simulink model "mult35x35_tb"  (Simulink 6.6)
settings: Solver=ode45  StartTime=0.0  StopTime=1000  RelTol=1e-3
undefined symbols (not defined in the file): A, B
libraries: xbsIndex_r4 x168, simulink x2, xbsCopyrightNotice_r4 x1
(part 2 of 2)

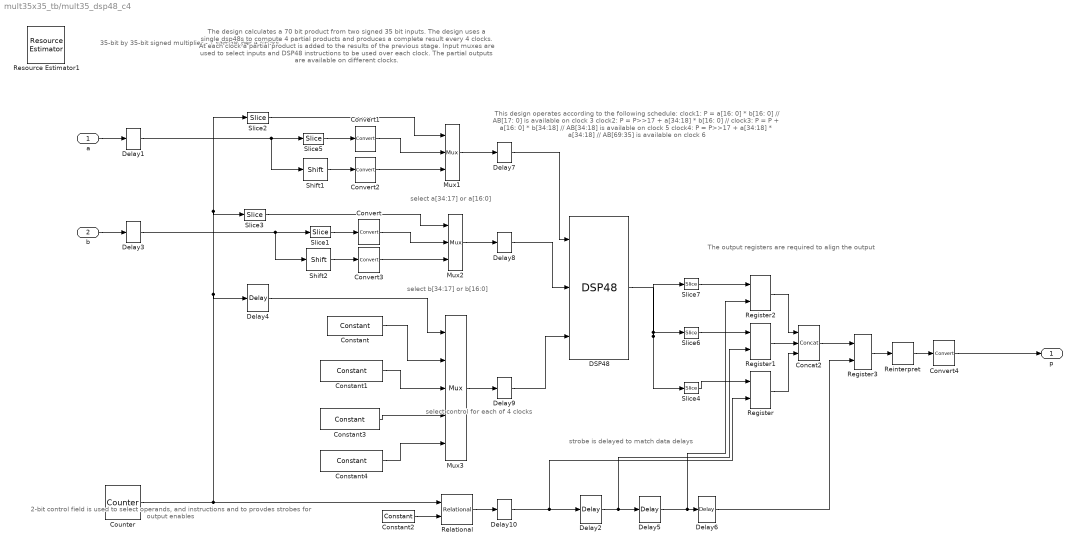
== system mult35x35_tb/mult35_dsp48_c4 ==
  note: select a[34:17] or a[16:0]
  note: 35-bit by 35-bit signed multiplier -
      | 1 sample per 4 clocks
  note: This design operates according to the following schedule:
      |
      | clock1: P =           a[16: 0] * b[16: 0] // AB[17: 0] is available on clock 3
      | clock2: P = P>>17  +  a[34:18] * b[16: 0] //
      | clock3: P = P      +  a[16: 0] * b[34:18] // AB[34:18] is available on clock 5
      | clock4: P = P>>17  +  a[34:18] * a[34:18] // AB[69:35] is available on clock 6
  note: select b[34:17] or b[16:0]
  note: select control for each of 4 clocks
  note: 2-bit control field is used to select operands,
      | and instructions and to provdes strobes for output enables
  note: The design calculates a 70 bit product from two signed 35 bit inputs.
      | The design uses a single  dsp48s to compute 4 partial products and produces a complete result every 4 clocks.
      | At each clock a partial product is added to the results of the previous stage. Input muxes are used to select inputs
      | and DSP48 instructions to be used over each clock. The partial outputs are available on different clocks.
  note: The output registers are required to align the output
  note: strobe is delayed to match data delays
  a : Inport
  b : Inport  Port=2
  Concat2 : xbsIndex_r4/Concat  num_inputs=3  dbl_ovrd=off  block_type=concat
      settings: block_version=VER_STRING_GOES_HERE
  Constant : xbsIndex_r4/Constant  arith_type=DSP48 Instruction  const=1  n_bits=1  bin_pt=0  explicit_period=off  period=1  equ=P=+A*B  opselect=A * B  inp2=PCIN>>17  opr=+  inp1=P  carry=CIN  dbl_ovrd=off  block_type=constant
      settings: block_version=VER_STRING_GOES_HERE
  Constant1 : xbsIndex_r4/Constant  arith_type=DSP48 Instruction  const=1  n_bits=1  bin_pt=0  explicit_period=off  period=1  equ=P=P>>17+(A*B)  opselect=Custom  inp2=P>>17  opr=+  inp1=A*B  carry=0  dbl_ovrd=off  block_type=constant
      settings: block_version=VER_STRING_GOES_HERE
  Constant2 : xbsIndex_r4/Constant  arith_type=Unsigned  const=3  n_bits=2  bin_pt=0  explicit_period=off  period=1  equ=P=C  opselect=C  inp2=PCIN>>17  opr=+  inp1=P  carry=CIN  dbl_ovrd=off  block_type=constant
      settings: block_version=VER_STRING_GOES_HERE
  Constant3 : xbsIndex_r4/Constant  arith_type=DSP48 Instruction  const=1  n_bits=1  bin_pt=0  explicit_period=off  period=1  equ=P=P+(A*B)  opselect=Custom  inp2=P  opr=+  inp1=A*B  carry=0  dbl_ovrd=off  block_type=constant
      settings: block_version=VER_STRING_GOES_HERE
  Constant4 : xbsIndex_r4/Constant  arith_type=DSP48 Instruction  const=1  n_bits=1  bin_pt=0  explicit_period=off  period=1  equ=P=P>>17+(A*B)  opselect=Custom  inp2=P>>17  opr=+  inp1=A*B  carry=0  dbl_ovrd=off  block_type=constant
      settings: block_version=VER_STRING_GOES_HERE
  Convert{,1..3} (4 alike) : xbsIndex_r4/Convert  arith_type="Signed  (2's comp)"  n_bits=18  bin_pt=0  quantization=Truncate  overflow=Wrap  latency=0  dbl_ovrd=off  pipeline=off  block_type=convert
      settings: infoedit=The input is presented at the output after quantization and overflow effects.<P><P>Hardware notes: Additional hardware is used when rounding or saturation is selected and output width is less than the input width.  xl_area=[0 0 0 0 0 0 0]  block_version=VER_STRING_GOES_HERE
  Convert4 : xbsIndex_r4/Convert  arith_type="Signed  (2's comp)"  n_bits=71  bin_pt=0  quantization=Truncate  overflow=Wrap  latency=0  dbl_ovrd=off  pipeline=off  block_type=convert
      settings: infoedit=The input is presented at the output after quantization and overflow effects.<P><P>Hardware notes: Additional hardware is used when rounding or saturation is selected and output width is less than the input width.  xl_area=[0 0 0 0 0 0 0]  block_version=VER_STRING_GOES_HERE
  Counter : xbsIndex_r4/Counter  cnt_type=Free Running  cnt_to=Inf  operation=Up  start_count=0  cnt_by_val=1  arith_type=Unsigned  n_bits=2  bin_pt=0  load_pin=off  rst=off  en=off  explicit_period=on  period=1  dbl_ovrd=off  use_behavioral_HDL=on  use_rpm=off  block_type=counter
      settings: infoedit="Configurable up, down and up/down counter.<P><P>Hardware notes: Free running counters are the least expensive in hardware.  A count limited counter is implemented by combining a counter with a comparator."  xl_area=[1 2 0 2 0 0 0]  block_version=VER_STRING_GOES_HERE
  DSP48 : xbsIndex_r4/DSP48  use_b=Direct from B Port  use_op=on  use_creg=off  use_pcin=off  use_pcout=off  use_bcout=off  rst_all=off  en_all=off  pipeline_a=1  pipeline_b=1  pipeline_c=on  pipeline_p=on  pipeline_mult=on  pipeline_opmode=on  pipeline_sub=on  pipeline_carryin=on  pipeline_carryinsel=on  rst_a=off  rst_b=off  rst_c=off  rst_mult=off  rst_p=off  rst_carry_in=off  rst_ctrl=off  en_a=off  en_b=off  en_c=off  en_mult=off  en_p=off  en_carry_in=off  en_ctrl=off  dbl_ovrd=off  use_synth_model=off  xl_useadderonly=off  block_type=dsp48
      settings: xl_use_area=on  xl_area=[0, 0, 0, 0, 0, 0, 0]  block_version=VER_STRING_GOES_HERE
  Delay{1,3..10} (9 alike) : xbsIndex_r4/Delay  en=off  latency=1  dbl_ovrd=off  reg_retiming=off  block_type=delay
      Delay1 settings: infoedit="Delay line having  configurable length.<P><P>Hardware notes: A delay line is a chain, each link of which is an SRL16 followed by a flip-flop. If register retiming is enabled, the delay line is a chain of flip-flops."  xl_area=[1 1 0 0 0 0 0]  block_version=VER_STRING_GOES_HERE
      Delay10 settings: infoedit="Delay line having  configurable length.<P><P>Hardware notes: A delay line is a chain, each link of which is an SRL16 followed by a flip-flop. If register retiming is enabled, the delay line is a chain of flip-flops."  xl_area=[1 1 0 0 0 0 0]  block_version=VER_STRING_GOES_HERE
      Delay3 settings: infoedit="Delay line having  configurable length.<P><P>Hardware notes: A delay line is a chain, each link of which is an SRL16 followed by a flip-flop. If register retiming is enabled, the delay line is a chain of flip-flops."  xl_area=[1 1 0 0 0 0 0]  block_version=VER_STRING_GOES_HERE
      Delay4 settings: infoedit="Delay line having  configurable length.<P><P>Hardware notes: A delay line is a chain, each link of which is an SRL16 followed by a flip-flop. If register retiming is enabled, the delay line is a chain of flip-flops."  xl_area=[1 2 0 0 0 0 0]  block_version=VER_STRING_GOES_HERE
      Delay5 settings: infoedit="Delay line having  configurable length.<P><P>Hardware notes: A delay line is a chain, each link of which is an SRL16 followed by a flip-flop. If register retiming is enabled, the delay line is a chain of flip-flops."  xl_area=[1 1 0 0 0 0 0]  block_version=VER_STRING_GOES_HERE
      Delay6 settings: infoedit="Delay line having  configurable length.<P><P>Hardware notes: A delay line is a chain, each link of which is an SRL16 followed by a flip-flop. If register retiming is enabled, the delay line is a chain of flip-flops."  xl_area=[1 1 0 0 0 0 0]  block_version=VER_STRING_GOES_HERE
      Delay7 settings: infoedit="Delay line having  configurable length.<P><P>Hardware notes: A delay line is a chain, each link of which is an SRL16 followed by a flip-flop. If register retiming is enabled, the delay line is a chain of flip-flops."  xl_area=[1 1 0 0 0 0 0]  block_version=VER_STRING_GOES_HERE
      Delay8 settings: infoedit="Delay line having  configurable length.<P><P>Hardware notes: A delay line is a chain, each link of which is an SRL16 followed by a flip-flop. If register retiming is enabled, the delay line is a chain of flip-flops."  xl_area=[1 1 0 0 0 0 0]  block_version=VER_STRING_GOES_HERE
      Delay9 settings: infoedit="Delay line having  configurable length.<P><P>Hardware notes: A delay line is a chain, each link of which is an SRL16 followed by a flip-flop. If register retiming is enabled, the delay line is a chain of flip-flops."  xl_area=[1 1 0 0 0 0 0]  block_version=VER_STRING_GOES_HERE
  Delay2 : xbsIndex_r4/Delay  en=off  latency=2  dbl_ovrd=off  reg_retiming=off  block_type=delay
      settings: infoedit="Delay line having  configurable length.<P><P>Hardware notes: A delay line is a chain, each link of which is an SRL16 followed by a flip-flop. If register retiming is enabled, the delay line is a chain of flip-flops."  xl_area=[1 1 0 1 0 0 0]  block_version=VER_STRING_GOES_HERE
  Mux1 : xbsIndex_r4/Mux  inputs=2  en=off  latency=0  precision=Full  arith_type=Unsigned  n_bits=48  bin_pt=0  quantization=Truncate  overflow=Wrap  dbl_ovrd=off  block_type=mux
      settings: xl_area=[9 0 0 18 0 0 0]  block_version=VER_STRING_GOES_HERE
  Mux2 : xbsIndex_r4/Mux  inputs=2  en=off  latency=0  precision=Full  arith_type=Unsigned  n_bits=48  bin_pt=0  quantization=Truncate  overflow=Wrap  dbl_ovrd=off  block_type=mux
      settings: xl_area=[9 0 0 18 0 0 0]  block_version=VER_STRING_GOES_HERE
  Mux3 : xbsIndex_r4/Mux  inputs=4  en=off  latency=0  precision=Full  arith_type=Unsigned  n_bits=48  bin_pt=0  quantization=Truncate  overflow=Wrap  dbl_ovrd=off  block_type=mux
      settings: xl_area=[11 0 0 22 0 0 0]  block_version=VER_STRING_GOES_HERE
  Register{,1..3} (4 alike) : xbsIndex_r4/Register  init=0  rst=off  en=on  dbl_ovrd=off  block_type=register
      Register settings: xl_area=[9 17 0 0 0 0 0]  block_version=VER_STRING_GOES_HERE
      Register1 settings: xl_area=[9 17 0 0 0 0 0]  block_version=VER_STRING_GOES_HERE
      Register2 settings: xl_area=[18 36 0 0 0 0 0]  block_version=VER_STRING_GOES_HERE
      Register3 settings: xl_area=[35 70 0 0 0 0 0]  block_version=VER_STRING_GOES_HERE
  Reinterpret : xbsIndex_r4/Reinterpret  force_arith_type=on  arith_type="Signed  (2's comp)"  force_bin_pt=on  bin_pt=0  block_type=cast
      settings: infoedit="Changes type of samples without altering their binary representation.<P><P>Hardware notes: In hardware this block costs nothing.<P><P>Example:  Suppose the input is 6 bits wide, signed, with 2 fractional bits, and the output is forced to unsigned with 0 fractional bits.  Then an input of -2.0 (1110.00 in binary 2's complement) becomes an output of 56 (111000 in binary)."  block_version=VER_STRING_GOES_HERE
  Relational : xbsIndex_r4/Relational  mode=a=b  en=off  latency=0  dbl_ovrd=off  block_type=relational
      settings: xl_area=[1 0 0 1 0 0 0]  block_version=VER_STRING_GOES_HERE
  Resource Estimator1 : xbsIndex_r4/Resource Estimator  Tag=resEstTag  Slices=896  FFs=1554  BRAMs=0  LUTs=775  IOBs=545  EBMs=8  TBUFs=0  xl_use_estimator_area=off  est_options=Estimate  xl_estimator_area=[896 1554 0 775 545 8 0]  mrp_directory=I:\sg48\src  simulink_period=1/16  block_type=resource_estimator
      settings: AttributesFormatString=Resource\nEstimator  block_version=9.2.00
  Shift1 : xbsIndex_r4/Shift  shift_dir=Right  shift_bits=17  en=off  latency=0  precision=Full  arith_type="Signed  (2's comp)"  n_bits=8  bin_pt=2  quantization=Truncate  overflow=Wrap  dbl_ovrd=off  block_type=shift
      settings: xl_area=[0 0 0 0 0 0 0]  block_version=VER_STRING_GOES_HERE
  Shift2 : xbsIndex_r4/Shift  shift_dir=Right  shift_bits=17  en=off  latency=0  precision=Full  arith_type="Signed  (2's comp)"  n_bits=8  bin_pt=2  quantization=Truncate  overflow=Wrap  dbl_ovrd=off  block_type=shift
      settings: xl_area=[0 0 0 0 0 0 0]  block_version=VER_STRING_GOES_HERE
  Slice{1,4..6} (4 alike) : xbsIndex_r4/Slice  nbits=17  boolean_output=off  mode=Lower Bit Location + Width  bit1=18  base1=LSB of Input  bit0=0  base0=LSB of Input  dbl_ovrd=off  block_type=slice
      settings: infoedit="Extracts a given range of bits from each input sample and presents it at the output.  The output type is ordinarily unsigned with binary point at zero, but can be Boolean when the slice is one bit wide.<P><P>Hardware notes: In hardware this block costs nothing."  block_version=VER_STRING_GOES_HERE
  Slice2 : xbsIndex_r4/Slice  nbits=1  boolean_output=off  mode=Lower Bit Location + Width  bit1=18  base1=LSB of Input  bit0=1  base0=LSB of Input  dbl_ovrd=off  block_type=slice
      settings: infoedit="Extracts a given range of bits from each input sample and presents it at the output.  The output type is ordinarily unsigned with binary point at zero, but can be Boolean when the slice is one bit wide.<P><P>Hardware notes: In hardware this block costs nothing."  block_version=VER_STRING_GOES_HERE
  Slice3 : xbsIndex_r4/Slice  nbits=1  boolean_output=off  mode=Lower Bit Location + Width  bit1=18  base1=LSB of Input  bit0=0  base0=LSB of Input  dbl_ovrd=off  block_type=slice
      settings: infoedit="Extracts a given range of bits from each input sample and presents it at the output.  The output type is ordinarily unsigned with binary point at zero, but can be Boolean when the slice is one bit wide.<P><P>Hardware notes: In hardware this block costs nothing."  block_version=VER_STRING_GOES_HERE
  Slice7 : xbsIndex_r4/Slice  nbits=36  boolean_output=off  mode=Lower Bit Location + Width  bit1=18  base1=LSB of Input  bit0=0  base0=LSB of Input  dbl_ovrd=off  block_type=slice
      settings: infoedit="Extracts a given range of bits from each input sample and presents it at the output.  The output type is ordinarily unsigned with binary point at zero, but can be Boolean when the slice is one bit wide.<P><P>Hardware notes: In hardware this block costs nothing."  block_version=VER_STRING_GOES_HERE
  p : Outport
  wires:
  a/1 -> Delay1/1
  b/1 -> Delay3/1
  Shift1/1 -> Convert2/1
  Slice5/1 -> Convert1/1
  Shift2/1 -> Convert3/1
  Slice1/1 -> Convert/1
  Slice3/1 -> Mux2/1
  Slice2/1 -> Mux1/1
  Slice4/1 -> Register/1
  Slice6/1 -> Register1/1
  Slice7/1 -> Register2/1
  Register/1 -> Concat2/3
  Register1/1 -> Concat2/2
  Register2/1 -> Concat2/1
  Convert4/1 -> p/1
  Constant2/1 -> Relational/2
  Relational/1 -> Delay10/1
  Delay2/1 -> Delay5/1, Register1/2
  Delay5/1 -> Register2/2, Delay6/1
  Concat2/1 -> Register3/1
  Register3/1 -> Reinterpret/1
  Delay6/1 -> Register3/2
  Convert1/1 -> Mux1/2
  Convert2/1 -> Mux1/3
  Convert3/1 -> Mux2/3
  Convert/1 -> Mux2/2
  Reinterpret/1 -> Convert4/1
  Mux3/1 -> Delay9/1
  Constant/1 -> Mux3/2
  Constant1/1 -> Mux3/3
  Constant3/1 -> Mux3/4
  Constant4/1 -> Mux3/5
  DSP48/1 -> Slice4/1, Slice6/1, Slice7/1
  Delay4/1 -> Mux3/1
  Counter/1 -> Relational/1, Delay4/1, Slice2/1, Slice3/1
  Mux1/1 -> Delay7/1
  Mux2/1 -> Delay8/1
  Delay7/1 -> DSP48/1
  Delay8/1 -> DSP48/2
  Delay9/1 -> DSP48/3
  Delay10/1 -> Delay2/1, Register/2
  Delay1/1 -> Shift1/1, Slice5/1
  Delay3/1 -> Slice1/1, Shift2/1

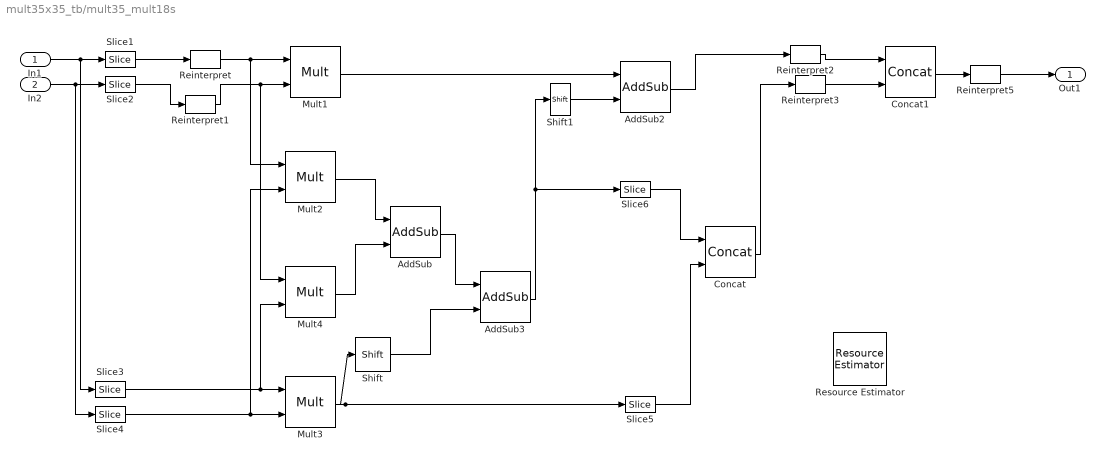
== system mult35x35_tb/mult35_mult18s ==
  In1 : Inport
  In2 : Inport  Port=2
  AddSub : xbsIndex_r4/AddSub  mode=Addition  use_carryin=off  use_carryout=off  en=off  latency=0  precision=Full  arith_type=Unsigned  n_bits=8  bin_pt=2  quantization=Truncate  overflow=Wrap  dbl_ovrd=off  use_behavioral_HDL=on  pipelined=off  use_rpm=off  block_type=addsub
      settings: xl_area=[18 0 0 35 0 0 0]  block_version=VER_STRING_GOES_HERE
  AddSub2 : xbsIndex_r4/AddSub  mode=Addition  use_carryin=off  use_carryout=off  en=off  latency=0  precision=Full  arith_type=Unsigned  n_bits=8  bin_pt=2  quantization=Truncate  overflow=Wrap  dbl_ovrd=off  use_behavioral_HDL=on  pipelined=off  use_rpm=off  block_type=addsub
      settings: xl_area=[19 0 0 37 0 0 0]  block_version=VER_STRING_GOES_HERE
  AddSub3 : xbsIndex_r4/AddSub  mode=Addition  use_carryin=off  use_carryout=off  en=off  latency=0  precision=Full  arith_type=Unsigned  n_bits=8  bin_pt=2  quantization=Truncate  overflow=Wrap  dbl_ovrd=off  use_behavioral_HDL=on  pipelined=off  use_rpm=off  block_type=addsub
      settings: xl_area=[19 0 0 36 0 0 0]  block_version=VER_STRING_GOES_HERE
  Concat : xbsIndex_r4/Concat  num_inputs=2  dbl_ovrd=off  block_type=concat
      settings: block_version=VER_STRING_GOES_HERE
  Concat1 : xbsIndex_r4/Concat  num_inputs=2  dbl_ovrd=off  block_type=concat
      settings: block_version=VER_STRING_GOES_HERE
  Mult{1..4} (4 alike) : xbsIndex_r4/Mult  precision=Full  arith_type="Signed  (2's comp)"  n_bits=8  bin_pt=2  quantization=Truncate  overflow=Wrap  en=off  latency=3  dbl_ovrd=off  use_behavioral_HDL=off  use_embedded=on  opt=Speed  optimum_pipeline=off  pipeline=on  use_rpm=on  placement_style=Rectangular shape  block_type=mult
      Mult1 settings: infoedit=Multiplies two values.<P><P>Hardware notes: To use the internal pipeline stage of the dedicated multiplier you must select 'Pipeline to Greatest Extent Possible'.  xl_area=[36 72 0 36 0 1 0]  block_version=VER_STRING_GOES_HERE
      Mult2 settings: infoedit=Multiplies two values.<P><P>Hardware notes: To use the internal pipeline stage of the dedicated multiplier you must select 'Pipeline to Greatest Extent Possible'.  xl_area=[36 70 0 35 0 1 0]  block_version=VER_STRING_GOES_HERE
      Mult3 settings: infoedit=Multiplies two values.<P><P>Hardware notes: To use the internal pipeline stage of the dedicated multiplier you must select 'Pipeline to Greatest Extent Possible'.  xl_area=[34 68 0 34 0 1 0]  block_version=VER_STRING_GOES_HERE
      Mult4 settings: infoedit=Multiplies two values.<P><P>Hardware notes: To use the internal pipeline stage of the dedicated multiplier you must select 'Pipeline to Greatest Extent Possible'.  xl_area=[36 70 0 35 0 1 0]  block_version=VER_STRING_GOES_HERE
  Reinterpret : xbsIndex_r4/Reinterpret  force_arith_type=on  arith_type="Signed  (2's comp)"  force_bin_pt=on  bin_pt=0  block_type=cast
      settings: infoedit="Changes type of samples without altering their binary representation.<P><P>Hardware notes: In hardware this block costs nothing.<P><P>Example:  Suppose the input is 6 bits wide, signed, with 2 fractional bits, and the output is forced to unsigned with 0 fractional bits.  Then an input of -2.0 (1110.00 in binary 2's complement) becomes an output of 56 (111000 in binary)."  block_version=VER_STRING_GOES_HERE
  Reinterpret1 : xbsIndex_r4/Reinterpret  force_arith_type=on  arith_type="Signed  (2's comp)"  force_bin_pt=on  bin_pt=0  block_type=cast
      settings: infoedit="Changes type of samples without altering their binary representation.<P><P>Hardware notes: In hardware this block costs nothing.<P><P>Example:  Suppose the input is 6 bits wide, signed, with 2 fractional bits, and the output is forced to unsigned with 0 fractional bits.  Then an input of -2.0 (1110.00 in binary 2's complement) becomes an output of 56 (111000 in binary)."  block_version=VER_STRING_GOES_HERE
  Reinterpret2 : xbsIndex_r4/Reinterpret  force_arith_type=on  arith_type=Unsigned  force_bin_pt=on  bin_pt=0  block_type=cast
      settings: infoedit="Changes type of samples without altering their binary representation.<P><P>Hardware notes: In hardware this block costs nothing.<P><P>Example:  Suppose the input is 6 bits wide, signed, with 2 fractional bits, and the output is forced to unsigned with 0 fractional bits.  Then an input of -2.0 (1110.00 in binary 2's complement) becomes an output of 56 (111000 in binary)."  block_version=VER_STRING_GOES_HERE
  Reinterpret3 : xbsIndex_r4/Reinterpret  force_arith_type=on  arith_type=Unsigned  force_bin_pt=on  bin_pt=0  block_type=cast
      settings: infoedit="Changes type of samples without altering their binary representation.<P><P>Hardware notes: In hardware this block costs nothing.<P><P>Example:  Suppose the input is 6 bits wide, signed, with 2 fractional bits, and the output is forced to unsigned with 0 fractional bits.  Then an input of -2.0 (1110.00 in binary 2's complement) becomes an output of 56 (111000 in binary)."  block_version=VER_STRING_GOES_HERE
  Reinterpret5 : xbsIndex_r4/Reinterpret  force_arith_type=on  arith_type="Signed  (2's comp)"  force_bin_pt=on  bin_pt=0  block_type=cast
      settings: infoedit="Changes type of samples without altering their binary representation.<P><P>Hardware notes: In hardware this block costs nothing.<P><P>Example:  Suppose the input is 6 bits wide, signed, with 2 fractional bits, and the output is forced to unsigned with 0 fractional bits.  Then an input of -2.0 (1110.00 in binary 2's complement) becomes an output of 56 (111000 in binary)."  block_version=VER_STRING_GOES_HERE
  Resource Estimator : xbsIndex_r4/Resource Estimator  Tag=resEstTag  Slices=198  FFs=280  BRAMs=0  LUTs=248  IOBs=0  EBMs=4  TBUFs=0  xl_use_estimator_area=off  est_options=Estimate  xl_estimator_area=[198 280 0 248 0 4 0]  mrp_directory=I:\sg48\src  simulink_period=1/16  block_type=resource_estimator
      settings: AttributesFormatString=Resource\nEstimator  block_version=9.2.00
  Shift : xbsIndex_r4/Shift  shift_dir=Right  shift_bits=17  en=off  latency=0  precision=Full  arith_type="Signed  (2's comp)"  n_bits=8  bin_pt=2  quantization=Truncate  overflow=Wrap  dbl_ovrd=off  block_type=shift
      settings: xl_area=[0 0 0 0 0 0 0]  block_version=VER_STRING_GOES_HERE
  Shift1 : xbsIndex_r4/Shift  shift_dir=Right  shift_bits=17  en=off  latency=0  precision=Full  arith_type="Signed  (2's comp)"  n_bits=8  bin_pt=2  quantization=Truncate  overflow=Wrap  dbl_ovrd=off  block_type=shift
      settings: xl_area=[0 0 0 0 0 0 0]  block_version=VER_STRING_GOES_HERE
  Slice1 : xbsIndex_r4/Slice  nbits=18  boolean_output=off  mode=Lower Bit Location + Width  bit1=18  base1=LSB of Input  bit0=17  base0=LSB of Input  dbl_ovrd=off  block_type=slice
      settings: infoedit="Extracts a given range of bits from each input sample and presents it at the output.  The output type is ordinarily unsigned with binary point at zero, but can be Boolean when the slice is one bit wide.<P><P>Hardware notes: In hardware this block costs nothing."  block_version=VER_STRING_GOES_HERE
  Slice2 : xbsIndex_r4/Slice  nbits=18  boolean_output=off  mode=Lower Bit Location + Width  bit1=18  base1=LSB of Input  bit0=17  base0=LSB of Input  dbl_ovrd=off  block_type=slice
      settings: infoedit="Extracts a given range of bits from each input sample and presents it at the output.  The output type is ordinarily unsigned with binary point at zero, but can be Boolean when the slice is one bit wide.<P><P>Hardware notes: In hardware this block costs nothing."  block_version=VER_STRING_GOES_HERE
  Slice{3..6} (4 alike) : xbsIndex_r4/Slice  nbits=17  boolean_output=off  mode=Lower Bit Location + Width  bit1=18  base1=LSB of Input  bit0=0  base0=LSB of Input  dbl_ovrd=off  block_type=slice
      settings: infoedit="Extracts a given range of bits from each input sample and presents it at the output.  The output type is ordinarily unsigned with binary point at zero, but can be Boolean when the slice is one bit wide.<P><P>Hardware notes: In hardware this block costs nothing."  block_version=VER_STRING_GOES_HERE
  Out1 : Outport
  wires:
  In1/1 -> Slice1/1, Slice3/1
  In2/1 -> Slice2/1, Slice4/1
  Mult3/1 -> Slice5/1, Shift/1
  Slice1/1 -> Reinterpret/1
  Slice2/1 -> Reinterpret1/1
  Slice3/1 -> Mult3/1, Mult4/2
  Slice4/1 -> Mult3/2, Mult2/2
  Mult1/1 -> AddSub2/1
  AddSub3/1 -> Shift1/1, Slice6/1
  Slice5/1 -> Concat/2
  Slice6/1 -> Concat/1
  AddSub2/1 -> Reinterpret2/1
  Concat/1 -> Reinterpret3/1
  Concat1/1 -> Reinterpret5/1
  Shift1/1 -> AddSub2/2
  Reinterpret/1 -> Mult1/1, Mult2/1
  Reinterpret1/1 -> Mult1/2, Mult4/1
  Reinterpret2/1 -> Concat1/1
  Reinterpret3/1 -> Concat1/2
  Mult2/1 -> AddSub/1
  Mult4/1 -> AddSub/2
  Shift/1 -> AddSub3/2
  AddSub/1 -> AddSub3/1
  Reinterpret5/1 -> Out1/1
